simulink model "Task_No6"  (R2023b)
settings: Solver=ode5  StartTime=0.0  StopTime=3600*24*7  FixedStep=1  RelTol=1e-3
InitFcn:
  | PARAMETERS;
StartFcn:
  | PARAMETERS;
values from neighbouring files (symbols this model uses):
  Conv_C_to_K = 273.15    [PARAMETERS.m]
  P_AC_AIR_FLOW = 1    [PARAMETERS.m]
  P_CP_AIR = 1012    [PARAMETERS.m]
  P_DENSITY_AIR = 1.2041    [PARAMETERS.m]
  P_DENSITY_BRICK = 2/(10^-3)    (= 2000)    [PARAMETERS.m]
  P_DENSITY_PUR = 150    [PARAMETERS.m]
  P_EM_GLASS = 0.94    [PARAMETERS.m]
  P_EM_WALL = 0.94    [PARAMETERS.m]
  P_HANDLER_AIR_FLOW = 0.1    [PARAMETERS.m]
  P_HUMAN = 100    [PARAMETERS.m]
  P_INIT_CO2 = 420    [PARAMETERS.m]
  P_M_HUMAN_CO2 = 0.02*P_DENSITY_CO2/3600    (= 1.1e-05)    [PARAMETERS.m]
  P_M_HUMAN_VAPOR = 500*10^-3/(24*3600)    (= 5.78703703704e-06)    [PARAMETERS.m]
  P_M_WINDOW_SPEC = 20    [PARAMETERS.m]
  P_THICK_BRICK = 0.175    [PARAMETERS.m]
  P_THICK_PUR = P_THICK_WALL - P_THICK_BRICK    (= 0.125)    [PARAMETERS.m]
  RH_INIT_BDR = 40    [PARAMETERS.m]
  T_BREATH = 34    [PARAMETERS.m]
  T_COOLER = 12    [PARAMETERS.m]
  T_HEATER = 50    [PARAMETERS.m]
  T_INIT_BDR = 22    [PARAMETERS.m]
  T_INIT_OUT = 2.9    [PARAMETERS.m]
  U_WALL = 0.32    [PARAMETERS.m]
  U_WINDOW = 3.0    (= 3)    [PARAMETERS.m]
undefined symbols (not defined in the file or in its folder): P_AREA_BATH, P_AREA_BDR1, P_AREA_BDR2, P_AREA_EAST_WALL_BATH, P_AREA_EAST_WALL_BDR2, P_AREA_EAST_WALL_KIT, P_AREA_HALL, P_AREA_KIT, P_AREA_LVR, P_AREA_NORTH_WALL_BATH, P_AREA_NORTH_WALL_BDR1, P_AREA_NORTH_WALL_BDR2, P_AREA_OUTER_WALL_BATH, P_AREA_OUTER_WALL_BDR1, P_AREA_OUTER_WALL_BDR2, P_AREA_OUTER_WALL_HALL, P_AREA_OUTER_WALL_KIT, P_AREA_OUTER_WALL_LVR, P_AREA_SOUTH_WALL_KIT, P_AREA_SOUTH_WALL_LVR, P_AREA_WALL_BATH_KIT, P_AREA_WALL_BDR1_BDR2, P_AREA_WALL_BDR1_HALL, P_AREA_WALL_BDR2_BATH, P_AREA_WALL_BDR2_HALL, P_AREA_WALL_HALL_BATH, P_AREA_WALL_HALL_LVR, P_AREA_WALL_LVR_KIT, P_AREA_WIN_BATH, P_AREA_WIN_BDRS, P_AREA_WIN_KIT, P_AREA_WIN_LVR, P_M_AIR_BATH, P_M_AIR_BDR1, P_M_AIR_BDR2, P_M_AIR_HALL, P_M_AIR_KIT, P_M_AIR_LVR, TBL_SOL_EAST_01, TBL_SOL_EAST_02, TBL_SOL_EAST_03, TBL_SOL_EAST_04, TBL_SOL_EAST_05, TBL_SOL_EAST_06, TBL_SOL_EAST_07, TBL_SOL_EAST_08, TBL_SOL_EAST_09, TBL_SOL_EAST_10, TBL_SOL_EAST_11, TBL_SOL_EAST_12, TBL_SOL_NORTH_01, TBL_SOL_NORTH_02, TBL_SOL_NORTH_03, TBL_SOL_NORTH_04, TBL_SOL_NORTH_05, TBL_SOL_NORTH_06, TBL_SOL_NORTH_07, TBL_SOL_NORTH_08, TBL_SOL_NORTH_09, TBL_SOL_NORTH_10 ... (+7)
libraries: fl_lib x166, nesl_utility x88, slpidlib x3
(part 1 of 5)
settings Model: Creator=Selim  LastModifiedBy=Selim

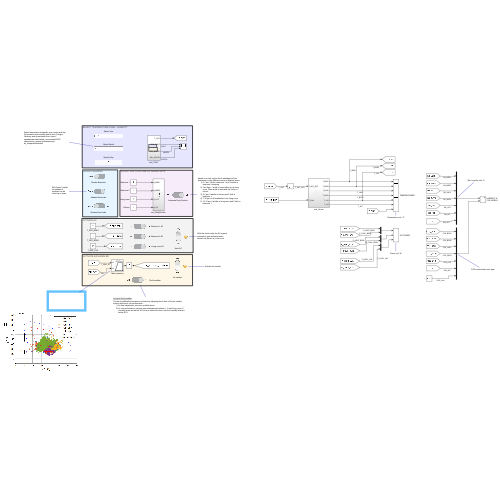
[thumbnail: Simulink's stored preview of the top-level diagram]
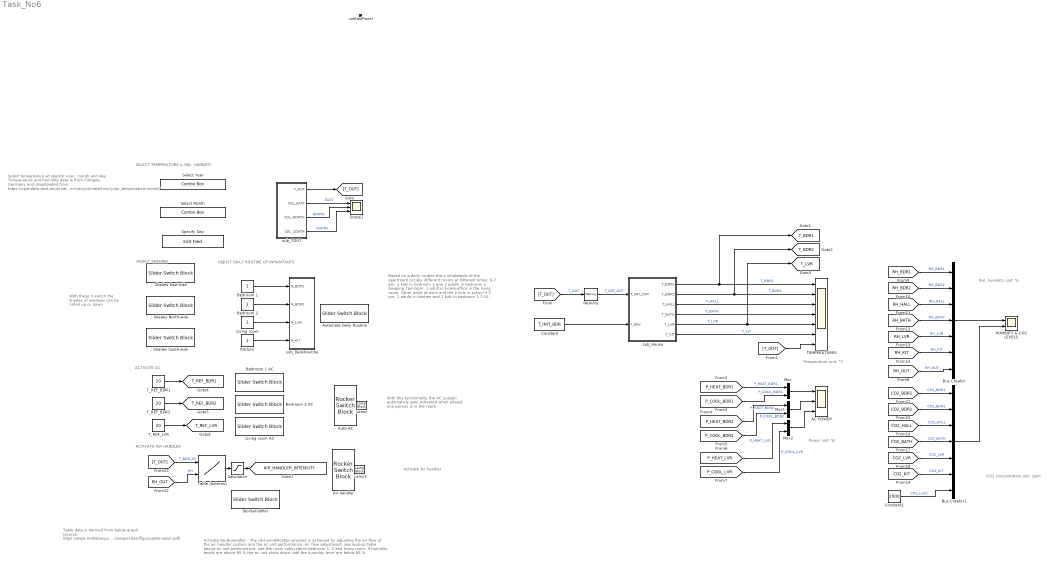
== system Task_No6 ==
  note: Table data is derived from below graph (source: https://www.matlabexpo.com/content/dam/mathworks/mathworks-dot-com/images/events/matlabexpo/de/2017/gebaude-und-anlagensimulation-mit-matlab-und-simulink-am-beispiel-des-ffg-projekts-saluh.pdf)
  note: Activate De-Humidifier :
      | The de-humidification process is achieved by adjusting the air flow of the air handler system and the ac unit performance.
      | Air flow adjustment: see look-up table above
      | Ac unit performance: see the room subsystems bedroom 1, 2 and living room. If humidity levels are above 85 % the ac unit shuts down until the humidity level are below 85 %.
  note: Activate Air handler
  note: Select temperature at specific year, month and day. Temperature and humidity data is from Cologne, Germany and downloaded from: https://opendata.dwd.de/climate_environment/CDC/observations_germany/climate/hourly/air_temperature/recent/
  note: ACTIVATE AIR HANDLER
  note: ACTIVATE AC
  note: ADJUST DAILY ROUTINE OF INHABITANTS
  note: ADJUST SHADING
  note: With these 3 switch the shades of windows can be rolled up or down
  note: CO2 concentration unit: ppm
  note: Rel. humidity unit: %
  note: Temperature unit: °C
  note: With this functionality the AC system automaticly gets activated when atleast one person is in the room
  note: SELECT TEMPERATURE & REL. HUMIDITY
  note: Based on a daily routine the 4 inhabitants of the apartment occupy different rooms at different times:
      | 0-7 am: 2 kids in bedroom 1 and 2 adults in bedroom 2 sleeping
      | 7am-5pm: 1 adult in home-office in the living room. Other adult at work and the 2 kids in school
      | 5-7 pm: 2 adults in kitchen and 2 kids in bedroom 1
      | 7-10 pm: all 4 inhabitants in the living room
      | 10-12 pm: 2 adults in living room and 2 kids in bedroom 1
  note: Power unit: W
  AC POWER : Scope  NumInputPorts=3
  Air handler : RockerSwitchBlock  LabelPosition=Hide
      settings: Values={{'Off', 'On'}, [0 1]}
  Auto-AC : RockerSwitchBlock  LabelPosition=Hide
      settings: Values={{'Off', 'On'}, [0 1]}
  Automate Daily Routine : SliderSwitchBlock  LabelPosition=Hide
      settings: Values={{'OFF', 'ON'}, [0 1]}
  Bedroom 1 : Constant
  Bedroom 1 AC : SliderSwitchBlock  LabelPosition=Hide
      settings: Values={{'OFF', 'ON'}, [0 1]}
  Bedroom 2 : Constant
  Bedroom 2 AC : SliderSwitchBlock  LabelPosition=Hide
      settings: Values={{'OFF', 'ON'}, [0 1]}
  Bus Creator : BusCreator  Inputs=7
  Bus Creator1 : BusCreator  Inputs=7
  Constant : Constant  Value=T_INIT_BDR
  Constant1 : Constant  Value=2000
  De-Humidifier : SliderSwitchBlock  LabelPosition=Hide
      settings: Values={{'OFF', 'ON'}, [0 1]}
  HUMIDITY & CO2 LEVELS : Scope  NumInputPorts=2
  Kitchen : Constant
  Lamp : LampBlock  LabelPosition=Hide
  Lamp1 : LampBlock  LabelPosition=Hide
  Living room : Constant
  Living room AC : SliderSwitchBlock  LabelPosition=Hide
      settings: Values={{'OFF', 'ON'}, [0 1]}
  Memory : Memory  InitialCondition=T_INIT_OUT
  Mux : Mux  Inputs=2
  Mux1 : Mux  Inputs=2
  Mux2 : Mux  Inputs=2
  Saturation : Saturate  UpperLimit=inf  LowerLimit=0
  Scope1 : Scope  NumInputPorts=3
  Select Month : ComboBox  LabelPosition=Hide  SelectedLabel=July
      settings: Values={{'January', 'February', 'March', 'April', 'May', 'June', 'July', 'August', 'September', 'Oktober', 'November', 'December'}, [1 2 3 4 5 6 7 8 9 10 11 12]}
  Select Year : ComboBox  LabelPosition=Hide  SelectedLabel=2023
      settings: Values={{'2022', '2023'}, [2022 2023]}
  Shades East-side : SliderSwitchBlock  LabelPosition=Hide
      settings: Values={{'Down', 'Up'}, [0 1]}
  Shades North-side : SliderSwitchBlock  LabelPosition=Hide
      settings: Values={{'Down', 'Up'}, [0 1]}
  Shades South-side : SliderSwitchBlock  LabelPosition=Hide
      settings: Values={{'Down', 'Up'}, [0 1]}
  Specify Day : EditField  LabelPosition=Hide  ShowInitialText=on  Alignment=Center
  TEMPERATURES : Scope  NumInputPorts=7
  T_REF_BDR1 : Constant  Value=20
  T_REF_BDR2 : Constant  Value=20
  T_REF_LVR : Constant  Value=20
  Table (exterior) : Lookup_n-D  BreakpointsForDimension1=[16;19;24;24.5]  BreakpointsForDimension2=[20;25;58;82]  Table=[0.5 0.5 0.5 0.5;0.5 1 1 0.5;0.5 1 1 0.5;0.5 0.5 0.5 0.5]  ExtrapMethod=Clip  InternalRulePriority=Speed  RndMeth=Simplest
      settings: InputPortMap=u0,u1
  sub_DailyRoutine : Subsystem
  sub_House : Subsystem
  sub_TOUT : Subsystem
  untitledPanel : Subsystem  Tag=HiddenForWebPanel  IsWebBlockPanel=on
  tag scope: AIR_HANDLER_INTENSITY=global, T_BDR1=global, T_BDR2=global, T_LVR=global, T_REF_BDR1=global, T_REF_BDR2=global, T_REF_LVR=global
  wires:
  Memory/1 -> sub_House/1(T_INIT_OUT)  "T_INIT_OUT"
  sub_House/1(T_BDR1) -> [T_BDR1], TEMPERATURES/1  "T_BDR1"
  [T_OUT] -> Memory/1  "T_OUT"
  [T_OUT] -> TEMPERATURES/7
  Constant/1 -> sub_House/2(T_ENV)
  sub_TOUT/1(T_OUT) -> [T_OUT]
  sub_House/2(T_BDR2) -> [T_BDR2], TEMPERATURES/2  "T_BDR2"
  sub_House/3(T_HALL) -> TEMPERATURES/3  "T_HALL"
  sub_House/4(T_BATH) -> TEMPERATURES/4  "T_BATH"
  sub_House/5(T_LVR) -> [T_LVR], TEMPERATURES/5  "T_LVR"
  sub_House/6(T_KIT) -> TEMPERATURES/6  "T_KIT"
  sub_TOUT/2(SOL_EAST) -> Scope1/1  "EAST"
  sub_TOUT/3(SOL_NORTH) -> Scope1/2  "NORTH"
  sub_TOUT/4(SOL_SOUTH) -> Scope1/3  "SOUTH"
  Bedroom 1/1 -> sub_DailyRoutine/1(N_BDR1)
  Bedroom 2/1 -> sub_DailyRoutine/2(N_BDR2)
  Living room/1 -> sub_DailyRoutine/3(N_LVR)
  Kitchen/1 -> sub_DailyRoutine/4(N_KIT)
  T_REF_BDR1/1 -> [T_REF_BDR1]
  T_REF_BDR2/1 -> [T_REF_BDR2]
  T_REF_LVR/1 -> [T_REF_LVR]
  Mux/1 -> AC POWER/1
  Mux1/1 -> AC POWER/2
  Mux2/1 -> AC POWER/3
  [P_HEAT_BDR1] -> Mux/1  "P_HEAT_BDR1"
  [P_COOL_BDR1] -> Mux/2  "P_COOL_BDR1"
  [P_HEAT_BDR2] -> Mux1/1  "P_HEAT_BDR2"
  [P_COOL_BDR2] -> Mux1/2  "P_COOL_BDR2"
  [P_HEAT_LVR] -> Mux2/1  "P_HEAT_LVR"
  [P_COOL_LVR] -> Mux2/2  "P_COOL_LVR"
  [RH_BDR1] -> Bus Creator/1  "RH_BDR1"
  [RH_BDR2] -> Bus Creator/2  "RH_BDR2"
  [RH_HALL] -> Bus Creator/3  "RH_HALL"
  [RH_BATH] -> Bus Creator/4  "RH_BATH"
  [RH_LVR] -> Bus Creator/5  "RH_LVR"
  [RH_KIT] -> Bus Creator/6  "RH_KIT"
  [RH_OUT] -> Bus Creator/7  "RH_OUT"
  [CO2_BDR1] -> Bus Creator1/1  "CO2_BDR1"
  [CO2_BDR2] -> Bus Creator1/2  "CO2_BDR2"
  [CO2_HALL] -> Bus Creator1/3  "CO2_HALL"
  [CO2_BATH] -> Bus Creator1/4  "CO2_BATH"
  [CO2_LVR] -> Bus Creator1/5  "CO2_LVR"
  [CO2_KIT] -> Bus Creator1/6  "CO2_KIT"
  Bus Creator/1 -> HUMIDITY & CO2 LEVELS/1
  Bus Creator1/1 -> HUMIDITY & CO2 LEVELS/2
  Constant1/1 -> Bus Creator1/7  "CO2_Limit"
  Table (exterior)/1 -> Saturation/1
  [T_OUT] -> Table (exterior)/1  "T_BDR_SC"
  [RH_OUT] -> Table (exterior)/2  "RH"
  Saturation/1 -> [AIR_HANDLER_INTENSITY]

== system Task_No6/sub_DailyRoutine ==
  N_BDR1 : Inport
  N_BDR2 : Inport  Port=2
  N_LVR : Inport  Port=3
  N_KIT : Inport  Port=4
  DAILY_ROUTINE_ON : Constant
  Memory1 : Memory
  Switch{,1..3} (4 alike) : Switch  Criteria=u2 > Threshold  SaturateOnIntegerOverflow=off  InputSameDT=off
  Time of day : MATLAB Function  TreatAsAtomicUnit=on
  tag scope: N_BDR1=global, N_BDR2=global, N_KIT=global, N_LVR=global
  wires:
  Switch1/1 -> [N_BDR2]
  Switch2/1 -> [N_LVR]
  Time of day/1(h) -> Memory1/1
  Memory1/1 -> Time of day/1("h ")
  Switch/1 -> [N_BDR1]
  Switch3/1 -> [N_KIT]
  Time of day/2(n_bdr1) -> Switch/1
  Time of day/3(n_bdr2) -> Switch1/1
  Time of day/4(n_lvr) -> Switch2/1
  Time of day/5(n_kit) -> Switch3/1
  DAILY_ROUTINE_ON/1 -> Switch3/2, Switch2/2, Switch1/2, Switch/2
  N_BDR1/1 -> Switch/3
  N_BDR2/1 -> Switch1/3
  N_LVR/1 -> Switch2/3
  N_KIT/1 -> Switch3/3

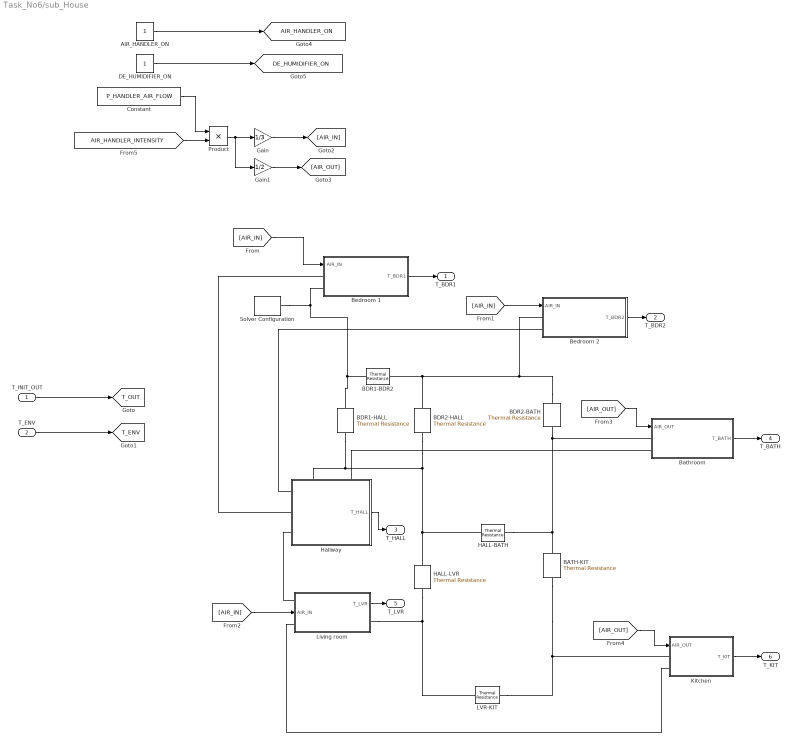
== system Task_No6/sub_House ==
  T_INIT_OUT : Inport
  T_ENV : Inport  Port=2
  AIR_HANDLER_ON : Constant
  BATH-KIT : fl_lib/Thermal/Thermal Elements/Thermal Resistance  resistance=1/(U_INNER_WALL_PC*P_AREA_WALL_BATH_KIT) K/W  T_specify=off  T_priority=None  T=0 K  T_nominal_specify=off  T_nominal_unit=K  T_nominal_value=1  Q_specify=off  Q_priority=None  Q=0 W  Q_nominal_specify=off  Q_nominal_unit=W  Q_nominal_value=1
  BDR1-BDR2 : fl_lib/Thermal/Thermal Elements/Thermal Resistance  resistance=1/(U_INNER_WALL_BR*P_AREA_WALL_BDR1_BDR2) K/W  T_specify=off  T_priority=None  T=0 K  T_nominal_specify=off  T_nominal_unit=K  T_nominal_value=1  Q_specify=off  Q_priority=None  Q=0 W  Q_nominal_specify=off  Q_nominal_unit=W  Q_nominal_value=1
  BDR1-HALL : fl_lib/Thermal/Thermal Elements/Thermal Resistance  resistance=1/(U_INNER_WALL_PC*P_AREA_WALL_BDR1_HALL) K/W  T_specify=off  T_priority=None  T=0 K  T_nominal_specify=off  T_nominal_unit=K  T_nominal_value=1  Q_specify=off  Q_priority=None  Q=0 W  Q_nominal_specify=off  Q_nominal_unit=W  Q_nominal_value=1
  BDR2-BATH : fl_lib/Thermal/Thermal Elements/Thermal Resistance  resistance=1/(U_INNER_WALL_PC*P_AREA_WALL_BDR2_BATH) K/W  T_specify=off  T_priority=None  T=0 K  T_nominal_specify=off  T_nominal_unit=K  T_nominal_value=1  Q_specify=off  Q_priority=None  Q=0 W  Q_nominal_specify=off  Q_nominal_unit=W  Q_nominal_value=1
  BDR2-HALL : fl_lib/Thermal/Thermal Elements/Thermal Resistance  resistance=1/(U_INNER_WALL_PC*P_AREA_WALL_BDR2_HALL) K/W  T_specify=off  T_priority=None  T=0 K  T_nominal_specify=off  T_nominal_unit=K  T_nominal_value=1  Q_specify=off  Q_priority=None  Q=0 W  Q_nominal_specify=off  Q_nominal_unit=W  Q_nominal_value=1
  Bathroom : Subsystem
  Bedroom 1 : Subsystem
  Bedroom 2 : Subsystem
  Constant : Constant  Value=P_HANDLER_AIR_FLOW
  DE_HUMIDIFIER_ON : Constant
  Gain : Gain  Gain=1/3
  Gain1 : Gain  Gain=1/2
  HALL-BATH : fl_lib/Thermal/Thermal Elements/Thermal Resistance  resistance=1/(U_INNER_WALL_BR*P_AREA_WALL_HALL_BATH) K/W  T_specify=off  T_priority=None  T=0 K  T_nominal_specify=off  T_nominal_unit=K  T_nominal_value=1  Q_specify=off  Q_priority=None  Q=0 W  Q_nominal_specify=off  Q_nominal_unit=W  Q_nominal_value=1
  HALL-LVR : fl_lib/Thermal/Thermal Elements/Thermal Resistance  resistance=1/(U_INNER_WALL_PC*P_AREA_WALL_HALL_LVR) K/W  T_specify=off  T_priority=None  T=0 K  T_nominal_specify=off  T_nominal_unit=K  T_nominal_value=1  Q_specify=off  Q_priority=None  Q=0 W  Q_nominal_specify=off  Q_nominal_unit=W  Q_nominal_value=1
  Hallway : Subsystem
      settings: PortSchema="{\"entries\":[{\"content\":{\"sides\":[{\"content\":{\"connectorIds\":[\"LConn1\",\"LConn2\",\"LConn3\"]},\"type\":\"ConnectorPlacement.EquallySpacedRectSide\",\"uuid\":\"489b9df6-19cb-4475-a274-302d4b8f34a0\"},{\"content\":{\"connectorIds\":[\"Out1\"],\"side\":\"RIGHT\"},\"type\":\"ConnectorPlacement.EquallySpacedRectSide\",\"uuid\":\"503e44aa-58ca-4784-9bf5-a317de849747\"},{\"content\":{\"connectorIds\":[\"LConn4\",\"LConn5\"],\"side\":\"TOP\"},\"type\":\"ConnectorPlacement.EquallySpacedRectSide\",\"uuid\":\"5734f698-8762-4391-9ecf-ea0e4ab42052\"}]},\"type\":\"ConnectorPlacement.EquallySpacedConnector\",\"uuid\":\"2aa354c6-d8ba-4f9b-b434-ff0d4333e4a9\"}],\"packageUris\":[\"http://schema.mathworks.com/mf0/Connector/R2020b\"],\"version\":\"1.0\"}"
  Kitchen : Subsystem
  LVR-KIT : fl_lib/Thermal/Thermal Elements/Thermal Resistance  resistance=1/(U_INNER_WALL_BR*P_AREA_WALL_LVR_KIT) K/W  T_specify=off  T_priority=None  T=0 K  T_nominal_specify=off  T_nominal_unit=K  T_nominal_value=1  Q_specify=off  Q_priority=None  Q=0 W  Q_nominal_specify=off  Q_nominal_unit=W  Q_nominal_value=1
  Living room : Subsystem
      settings: PortSchema="{\"entries\":[{\"content\":{\"sides\":[{\"content\":{\"connectorIds\":[\"LConn1\",\"In1\",\"LConn2\"]},\"type\":\"ConnectorPlacement.EquallySpacedRectSide\",\"uuid\":\"f71185e0-26fc-428d-a49e-eba48eb4716b\"},{\"content\":{\"connectorIds\":[\"Out1\",\"RConn1\"],\"side\":\"RIGHT\"},\"type\":\"ConnectorPlacement.EquallySpacedRectSide\",\"uuid\":\"b5ccd292-c29d-4ca4-a01f-fb6127cce0f9\"},{\"content\":{\"side\":\"TOP\"},\"type\":\"ConnectorPlacement.EquallySpacedRectSide\",\"uuid\":\"45f0e2e7-39cb-4c88-b766-6fb6aae0cec8\"}]},\"type\":\"ConnectorPlacement.EquallySpacedConnector\",\"uuid\":\"6a8451ab-eb03-49e5-afa1-3415116fa991\"}],\"packageUris\":[\"http://schema.mathworks.com/mf0/Connector/R2020b\"],\"version\":\"1.0\"}"
  Product : Product
  Solver Configuration : nesl_utility/Solver Configuration  PhysicalDomain=network_engine_domain  SubClassName=solver  LeftPortType=input  RightPortType=generic  Tones=[]  Harmonics=[]  SimulateNoise=off  Profile=off  UseLocalSampling=off  EnableSwitchedLinearOptims=on  FrequencyDomain=off  UseCCode=off  RelTol=0.001  AbsTol=0.001  MinStep=1e-09  ToWorkspace=off  RevertToSquareIcSolve=off  NumHomotopyIterations=100  PhasorMode=off  PhasorModeNumHarmonics=1  ConsistencySolver=NEWTON_XTOL_AFTER_FTOL  IndexReductionMethod=DerivativeReplacement  DoDC=off  ResidualTolerance=1e-09  ConsistencyTolSource=GLOBAL  ConsistencyAbsTol=0.001  ConsistencyRelTol=0.001  ConsistencyTolFactor=0.001  UseLocalSolver=on  LocalSolverChoice=NE_BACKWARD_EULER_ADVANCER  ResolveIndetEquations=on  FunctionEvalNumThread=1  LocalSolverSampleTime=1  DoFixedCost=on  MaxNonlinIter=3  MaxModeIter=2  ComputeImpulses=off  ImpulseIterations=2  LinearAlgebra=auto  LinearAlgebraNumThread=0  EquationFormulation=NE_TIME_EF  DelaysMemoryBudget=1024  AutomaticFiltering=on  FilteringTimeConstant=0.001  PartitionStorageMethod=AS_NEEDED  PartitionMemoryBudget=1024  PartitionMethod=ROBUST  MultibodyUseLocalSolver=off  MultibodyLocalSolverChoice=ODE1  MultibodyLocalSolverSampleTime=0.001
  T_BDR1 : Outport
  T_BDR2 : Outport  Port=2
  T_HALL : Outport  Port=3
  T_BATH : Outport  Port=4
  T_LVR : Outport  Port=5
  T_KIT : Outport  Port=6
  tag scope: AIR_HANDLER_ON=global, DE_HUMIDIFIER_ON=global, T_ENV=global, T_OUT=global
  wires:
  T_INIT_OUT/1 -> [T_OUT]
  T_ENV/1 -> [T_ENV]
  Bedroom 1/1(T_BDR1) -> T_BDR1/1
  Bedroom 2/1(T_BDR2) -> T_BDR2/1
  Hallway/1(T_HALL) -> T_HALL/1
  Living room/1(T_LVR) -> T_LVR/1
  Bathroom/1(T_BATH) -> T_BATH/1
  Kitchen/1(T_KIT) -> T_KIT/1
  Constant/1 -> Product/1
  Gain/1 -> [AIR_IN]
  [AIR_IN] -> Bedroom 1/1(AIR_IN)
  [AIR_IN] -> Bedroom 2/1(AIR_IN)
  [AIR_IN] -> Living room/1(AIR_IN)
  Gain1/1 -> [AIR_OUT]
  [AIR_OUT] -> Bathroom/1(AIR_OUT)
  [AIR_OUT] -> Kitchen/1(AIR_OUT)
  AIR_HANDLER_ON/1 -> [AIR_HANDLER_ON]
  [AIR_HANDLER_INTENSITY] -> Product/2
  Product/1 -> Gain/1, Gain1/1
  DE_HUMIDIFIER_ON/1 -> [DE_HUMIDIFIER_ON]
  connections:
  Solver Configuration/RConn1 -- BDR1-HALL/LConn1 -- BDR1-BDR2/RConn1 -- Bedroom 1/LConn2
  BDR2-BATH/LConn1 -- Bedroom 2/LConn1 -- BDR2-HALL/LConn1 -- BDR1-BDR2/LConn1
  BDR2-BATH/RConn1 -- HALL-BATH/LConn1 -- BATH-KIT/LConn1 -- Bathroom/LConn1
  HALL-LVR/RConn1 -- LVR-KIT/RConn1 -- Living room/RConn1
  BDR1-HALL/RConn1 -- HALL-LVR/LConn1 -- HALL-BATH/RConn1 -- BDR2-HALL/RConn1 -- Hallway/LConn4
  Hallway/LConn2 -- Bedroom 1/LConn1
  Hallway/LConn1 -- Bedroom 2/LConn2
  Living room/LConn1 -- Hallway/LConn3
  Hallway/LConn5 -- Bathroom/LConn2
  BATH-KIT/RConn1 -- LVR-KIT/LConn1 -- Kitchen/LConn1
  Kitchen/LConn2 -- Living room/LConn2

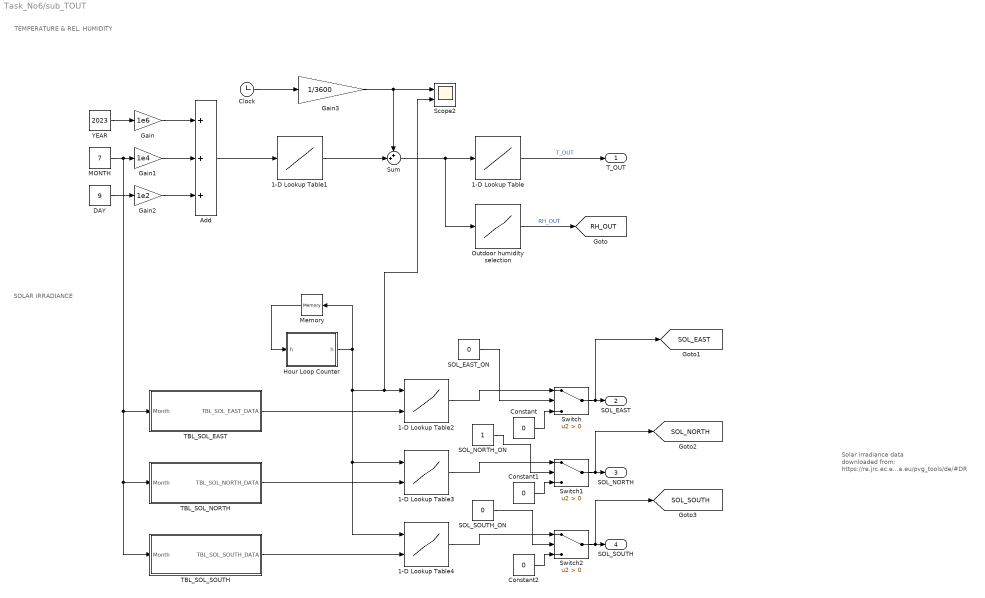
== system Task_No6/sub_TOUT ==
  note: Solar irradiance data downloaded from: https://re.jrc.ec.europa.eu/pvg_tools/de/#DR
  note: SOLAR IRRADIANCE
  note: TEMPERATURE & REL. HUMIDITY
  1-D Lookup Table : Lookup_n-D  NumberOfTableDimensions=1  BreakpointsForDimension1=TBL_TEMP.DATE_sec  Table=TBL_TEMP.T_C  InternalRulePriority=Speed  RndMeth=Simplest
  1-D Lookup Table1 : Lookup_n-D  NumberOfTableDimensions=1  BreakpointsForDimension1=TBL_TEMP.DATE_yyyymmddhh  Table=TBL_TEMP.DATE_sec  InternalRulePriority=Speed  RndMeth=Simplest
  1-D Lookup Table2 : Lookup_n-D  NumberOfTableDimensions=1  BreakpointsForDimension1=0:1:23  TableSource=Input port  Table=tanh([-5:5])  InternalRulePriority=Speed  RndMeth=Simplest
      settings: InputPortMap=u0,p221
  1-D Lookup Table3 : Lookup_n-D  NumberOfTableDimensions=1  BreakpointsForDimension1=0:1:23  TableSource=Input port  Table=tanh([-5:5])  InternalRulePriority=Speed  RndMeth=Simplest
      settings: InputPortMap=u0,p221
  1-D Lookup Table4 : Lookup_n-D  NumberOfTableDimensions=1  BreakpointsForDimension1=0:1:23  TableSource=Input port  Table=tanh([-5:5])  InternalRulePriority=Speed  RndMeth=Simplest
      settings: InputPortMap=u0,p221
  Add : Sum  Inputs=+++
  Clock : Clock
  Constant : Constant  Value=0
  Constant1 : Constant  Value=0
  Constant2 : Constant  Value=0
  DAY : Constant  Value=9
  Gain : Gain  Gain=1e6
  Gain1 : Gain  Gain=1e4
  Gain2 : Gain  Gain=1e2
  Gain3 : Gain  Gain=1/3600
  Hour Loop Counter : MATLAB Function  TreatAsAtomicUnit=on
  MONTH : Constant  Value=7
  Memory : Memory
  Outdoor humidity selection : Lookup_n-D  NumberOfTableDimensions=1  BreakpointsForDimension1=TBL_TEMP.DATE_sec  Table=TBL_TEMP.RM_p100  InternalRulePriority=Speed  RndMeth=Simplest
  SOL_EAST_ON : Constant  Value=0
  SOL_NORTH_ON : Constant
  SOL_SOUTH_ON : Constant  Value=0
  Scope2 : Scope  NumInputPorts=2
  Sum : Sum  Inputs=++|
  Switch : Switch  Criteria=u2 > Threshold  SaturateOnIntegerOverflow=off  InputSameDT=off
  Switch1 : Switch  Criteria=u2 > Threshold  SaturateOnIntegerOverflow=off  InputSameDT=off
  Switch2 : Switch  Criteria=u2 > Threshold  SaturateOnIntegerOverflow=off  InputSameDT=off
  TBL_SOL_EAST : Subsystem
  TBL_SOL_NORTH : Subsystem
  TBL_SOL_SOUTH : Subsystem
  YEAR : Constant  Value=2023
  T_OUT : Outport
  SOL_EAST : Outport  Port=2
  SOL_NORTH : Outport  Port=3
  SOL_SOUTH : Outport  Port=4
  tag scope: RH_OUT=global, SOL_EAST=global, SOL_NORTH=global, SOL_SOUTH=global
  wires:
  Gain1/1 -> Add/2
  MONTH/1 -> TBL_SOL_SOUTH/1(Month), TBL_SOL_NORTH/1(Month), TBL_SOL_EAST/1(Month), Gain1/1
  Clock/1 -> Gain3/1
  1-D Lookup Table1/1 -> Sum/2
  Add/1 -> 1-D Lookup Table1/1
  YEAR/1 -> Gain/1
  Gain/1 -> Add/1
  Gain3/1 -> Scope2/1, Sum/1
  Sum/1 -> Outdoor humidity selection/1, 1-D Lookup Table/1
  Gain2/1 -> Add/3
  DAY/1 -> Gain2/1
  1-D Lookup Table/1 -> T_OUT/1  "T_OUT"
  Hour Loop Counter/1(h) -> 1-D Lookup Table4/1, 1-D Lookup Table3/1, Scope2/2, 1-D Lookup Table2/1, Memory/1
  Memory/1 -> Hour Loop Counter/1("h ")
  Switch/1 -> [SOL_EAST], SOL_EAST/1
  TBL_SOL_EAST/1(TBL_SOL_EAST_DATA) -> 1-D Lookup Table2/2
  TBL_SOL_NORTH/1(TBL_SOL_NORTH_DATA) -> 1-D Lookup Table3/2
  TBL_SOL_SOUTH/1(TBL_SOL_SOUTH_DATA) -> 1-D Lookup Table4/2
  Switch1/1 -> [SOL_NORTH], SOL_NORTH/1
  Switch2/1 -> [SOL_SOUTH], SOL_SOUTH/1
  1-D Lookup Table2/1 -> Switch/1
  1-D Lookup Table3/1 -> Switch1/1
  1-D Lookup Table4/1 -> Switch2/1
  SOL_EAST_ON/1 -> Switch/2
  Constant/1 -> Switch/3
  Constant1/1 -> Switch1/3
  Constant2/1 -> Switch2/3
  SOL_NORTH_ON/1 -> Switch1/2
  SOL_SOUTH_ON/1 -> Switch2/2
  Outdoor humidity selection/1 -> [RH_OUT]  "RH_OUT"

== system Task_No6/untitledPanel ==
  Radio Button : RadioButtonGroup  Tag=HiddenForWebPanel  PanelInfo="{\"addnFilesFolder\":\"\",\"height\":230,\"includeDebugPackages\":false,\"left\":18,\"outputFolder\":\"\",\"panelId\":\"panelId-a10107d6-1e7d-451d-956e-0df6eada92c1\",\"popoutMode\":\"\",\"standaloneTitle\":\"\",\"top\":18,\"type\":\"panelChild\",\"version\":\"2019b\",\"width\":270,\"zIndex\":1500002}"  SelectedLabel=Label3  ButtonGroupName=Group
      settings: Values={{'Label1', 'Label2', 'Label3'}, [0 1 2]}
  panelInfo : PanelWebBlock  Tag=HiddenForWebPanel  PanelInfo="{\"addnFilesFolder\":\"\",\"compacted\":false,\"height\":270,\"includeDebugPackages\":false,\"isActiveTab\":true,\"left\":296,\"name\":\"Panel\",\"outputFolder\":\"\",\"panelId\":\"panelId-a10107d6-1e7d-451d-956e-0df6eada92c1\",\"popoutData\":{\"height\":334,\"left\":361,\"maximized\":false,\"top\":306,\"width\":324},\"popoutMode\":\"windowHidden\",\"standaloneTitle\":\"\",\"tabIndex\":0,\"tabbedSetId\":\"tabbedSet8433950298\",\"top\":135,\"type\":\"panel\",\"version\":\"2019b\",\"visible\":true,\"width\":310,\"zIndex\":1500002}"

== system Task_No6/sub_House/Bathroom ==
  AIR_OUT : Inport
  Bathroom : Subsystem
  MA Bathroom : Subsystem
  Product : Product
  Conn1 : PMIOPort  Side=Left
  HALL-BATH : PMIOPort  Port=2  Side=Left
  T_BATH : Outport
  wires:
  AIR_OUT/1 -> Product/1
  Bathroom/1(T_BATH) -> T_BATH/1
  [AIR_HANDLER_ON] -> Product/2
  Product/1 -> MA Bathroom/1(In1)
  connections:
  MA Bathroom/RConn1 -- Conn1/RConn1 -- Bathroom/LConn1
  HALL-BATH/RConn1 -- MA Bathroom/LConn1

== system Task_No6/sub_House/Bedroom 1 ==
  AIR_IN : Inport
  Bedroom 1 : Subsystem
  MA Bedroom 1 : Subsystem
  Product : Product
  BDR1-HALL : PMIOPort  Side=Left
  Conn1 : PMIOPort  Port=2  Side=Left
  T_BDR1 : Outport
  wires:
  AIR_IN/1 -> Product/1
  Bedroom 1/1(T_BDR1) -> T_BDR1/1
  Product/1 -> MA Bedroom 1/1(In1)
  [AIR_HANDLER_ON] -> Product/2
  connections:
  MA Bedroom 1/RConn1 -- Conn1/RConn1 -- Bedroom 1/LConn1
  BDR1-HALL/RConn1 -- MA Bedroom 1/LConn1

== system Task_No6/sub_House/Bedroom 2 ==
  AIR_IN : Inport
  Bedroom 2 : Subsystem
  MA Bedroom 2 : Subsystem
  Product : Product
  Conn1 : PMIOPort  Side=Left
  BDR2-HALL : PMIOPort  Port=2  Side=Left
  T_BDR2 : Outport
  wires:
  Bedroom 2/1(T_BDR2) -> T_BDR2/1
  AIR_IN/1 -> Product/1
  [AIR_HANDLER_ON] -> Product/2
  Product/1 -> MA Bedroom 2/1(In1)
  connections:
  BDR2-HALL/RConn1 -- MA Bedroom 2/LConn1
  MA Bedroom 2/RConn1 -- Conn1/RConn1 -- Bedroom 2/LConn1

== system Task_No6/sub_House/Hallway ==
  Hallway : Subsystem
  MA Hallway : Subsystem
  BDR2-HALL : PMIOPort  Side=Left
  BDR1-HALL : PMIOPort  Port=2  Side=Left
  LVR-HALL : PMIOPort  Port=3  Side=Left
  Conn4 : PMIOPort  Port=4  Side=Left
  HALL-BATH : PMIOPort  Port=5  Side=Left
  T_HALL : Outport
  wires:
  Hallway/1(T_HALL) -> T_HALL/1
  connections:
  MA Hallway/LConn4 -- HALL-BATH/RConn1
  Conn4/RConn1 -- MA Hallway/RConn1 -- Hallway/LConn1
  MA Hallway/LConn2 -- BDR1-HALL/RConn1
  MA Hallway/LConn1 -- BDR2-HALL/RConn1
  LVR-HALL/RConn1 -- MA Hallway/LConn3

== system Task_No6/sub_House/Kitchen ==
  AIR_OUT : Inport
  Kitchen : Subsystem
  MA Kitchen : Subsystem
  Product : Product
  Conn1 : PMIOPort  Side=Left
  LVR-KIT : PMIOPort  Port=2  Side=Left
  T_KIT : Outport
  wires:
  AIR_OUT/1 -> Product/1
  Kitchen/1(T_KIT) -> T_KIT/1
  Product/1 -> MA Kitchen/1(In1)
  [AIR_HANDLER_ON] -> Product/2
  connections:
  MA Kitchen/LConn1 -- LVR-KIT/RConn1
  Conn1/RConn1 -- MA Kitchen/RConn1 -- Kitchen/LConn1

== system Task_No6/sub_House/Living room ==
  AIR_IN : Inport
  Living Room : Subsystem
  MA Living Room : Subsystem
  Product : Product
  LVR-HALL : PMIOPort  Side=Left
  LVR-KIT : PMIOPort  Port=2  Side=Left
  Conn2 : PMIOPort  Port=3  Side=Right
  T_LVR : Outport
  wires:
  AIR_IN/1 -> Product/1
  Living Room/1(T_LVR) -> T_LVR/1
  [AIR_HANDLER_ON] -> Product/2
  Product/1 -> MA Living Room/1(In1)
  connections:
  LVR-KIT/RConn1 -- MA Living Room/LConn2
  Conn2/RConn1 -- Living Room/LConn1 -- MA Living Room/RConn1
  MA Living Room/LConn1 -- LVR-HALL/RConn1

== system Task_No6/sub_TOUT/TBL_SOL_EAST ==
  Month : Inport
  Constant : Constant  Value=TBL_SOL_EAST_01.G
  Constant1 : Constant  Value=TBL_SOL_EAST_02.G
  Constant10 : Constant  Value=TBL_SOL_EAST_11.G
  Constant11 : Constant  Value=TBL_SOL_EAST_12.G
  Constant2 : Constant  Value=TBL_SOL_EAST_03.G
  Constant3 : Constant  Value=TBL_SOL_EAST_04.G
  Constant4 : Constant  Value=TBL_SOL_EAST_05.G
  Constant5 : Constant  Value=TBL_SOL_EAST_06.G
  Constant6 : Constant  Value=TBL_SOL_EAST_07.G
  Constant7 : Constant  Value=TBL_SOL_EAST_08.G
  Constant8 : Constant  Value=TBL_SOL_EAST_09.G
  Constant9 : Constant  Value=TBL_SOL_EAST_10.G
  Multiport Switch : MultiPortSwitch  Inputs=12  SaturateOnIntegerOverflow=off  InputSameDT=off
  TBL_SOL_EAST_DATA : Outport
  wires:
  Constant1/1 -> Multiport Switch/3
  Constant5/1 -> Multiport Switch/7
  Constant6/1 -> Multiport Switch/8
  Constant3/1 -> Multiport Switch/5
  Multiport Switch/1 -> TBL_SOL_EAST_DATA/1
  Constant11/1 -> Multiport Switch/13
  Constant/1 -> Multiport Switch/2
  Constant2/1 -> Multiport Switch/4
  Constant7/1 -> Multiport Switch/9
  Constant4/1 -> Multiport Switch/6
  Constant10/1 -> Multiport Switch/12
  Constant9/1 -> Multiport Switch/11
  Constant8/1 -> Multiport Switch/10
  Month/1 -> Multiport Switch/1

== system Task_No6/sub_TOUT/TBL_SOL_NORTH ==
  Month : Inport
  Constant : Constant  Value=TBL_SOL_NORTH_01.G
  Constant1 : Constant  Value=TBL_SOL_NORTH_02.G
  Constant10 : Constant  Value=TBL_SOL_NORTH_11.G
  Constant11 : Constant  Value=TBL_SOL_NORTH_12.G
  Constant2 : Constant  Value=TBL_SOL_NORTH_03.G
  Constant3 : Constant  Value=TBL_SOL_NORTH_04.G
  Constant4 : Constant  Value=TBL_SOL_NORTH_05.G
  Constant5 : Constant  Value=TBL_SOL_NORTH_06.G
  Constant6 : Constant  Value=TBL_SOL_NORTH_07.G
  Constant7 : Constant  Value=TBL_SOL_NORTH_08.G
  Constant8 : Constant  Value=TBL_SOL_NORTH_09.G
  Constant9 : Constant  Value=TBL_SOL_NORTH_10.G
  Multiport Switch : MultiPortSwitch  Inputs=12  SaturateOnIntegerOverflow=off  InputSameDT=off
  TBL_SOL_NORTH_DATA : Outport
  wires:
  Month/1 -> Multiport Switch/1
  Constant8/1 -> Multiport Switch/10
  Constant9/1 -> Multiport Switch/11
  Constant10/1 -> Multiport Switch/12
  Constant4/1 -> Multiport Switch/6
  Constant7/1 -> Multiport Switch/9
  Constant2/1 -> Multiport Switch/4
  Constant/1 -> Multiport Switch/2
  Constant11/1 -> Multiport Switch/13
  Multiport Switch/1 -> TBL_SOL_NORTH_DATA/1
  Constant3/1 -> Multiport Switch/5
  Constant6/1 -> Multiport Switch/8
  Constant5/1 -> Multiport Switch/7
  Constant1/1 -> Multiport Switch/3

== system Task_No6/sub_TOUT/TBL_SOL_SOUTH ==
  Month : Inport
  Constant{,1..11} (12 alike) : Constant  Value=TBL_SOL_SOUTH_01.G
  Multiport Switch : MultiPortSwitch  Inputs=12  SaturateOnIntegerOverflow=off  InputSameDT=off
  TBL_SOL_SOUTH_DATA : Outport
  wires:
  Constant1/1 -> Multiport Switch/3
  Constant5/1 -> Multiport Switch/7
  Constant6/1 -> Multiport Switch/8
  Constant3/1 -> Multiport Switch/5
  Multiport Switch/1 -> TBL_SOL_SOUTH_DATA/1
  Constant11/1 -> Multiport Switch/13
  Constant/1 -> Multiport Switch/2
  Constant2/1 -> Multiport Switch/4
  Constant7/1 -> Multiport Switch/9
  Constant4/1 -> Multiport Switch/6
  Constant10/1 -> Multiport Switch/12
  Constant9/1 -> Multiport Switch/11
  Constant8/1 -> Multiport Switch/10
  Month/1 -> Multiport Switch/1

== system Task_No6/sub_House/Bathroom/Bathroom ==
  Ceiling & Floor (Bath<->Above & Below) : Subsystem
  Inside Enivornment Temperature : Subsystem
      settings: PortSchema="{\"entries\":[{\"content\":{\"sides\":[{\"content\":{\"connectorIds\":[\"LConn1\"]},\"type\":\"ConnectorPlacement.EquallySpacedRectSide\",\"uuid\":\"d7207a88-d4d1-4eb1-8525-bfbf38cfed80\"},{\"content\":{\"connectorIds\":[\"In1\"],\"side\":\"RIGHT\"},\"type\":\"ConnectorPlacement.EquallySpacedRectSide\",\"uuid\":\"a5beddf3-616c-4e89-970e-855bf6dc3854\"},{\"content\":{\"side\":\"TOP\"},\"type\":\"ConnectorPlacement.EquallySpacedRectSide\",\"uuid\":\"3f9b2b25-be8a-4286-a049-e39ed58f5b46\"}]},\"type\":\"ConnectorPlacement.EquallySpacedConnector\",\"uuid\":\"525311df-b3f4-411a-b576-8112a1b0b63b\"}],\"packageUris\":[\"http://schema.mathworks.com/mf0/Connector/R2020b\"],\"version\":\"1.0\"}"
  Outside Temperature : Subsystem
      settings: PortSchema="{\"entries\":[{\"content\":{\"sides\":[{\"content\":{\"connectorIds\":[\"LConn1\"]},\"type\":\"ConnectorPlacement.EquallySpacedRectSide\",\"uuid\":\"d7207a88-d4d1-4eb1-8525-bfbf38cfed80\"},{\"content\":{\"connectorIds\":[\"In1\"],\"side\":\"RIGHT\"},\"type\":\"ConnectorPlacement.EquallySpacedRectSide\",\"uuid\":\"a5beddf3-616c-4e89-970e-855bf6dc3854\"},{\"content\":{\"side\":\"TOP\"},\"type\":\"ConnectorPlacement.EquallySpacedRectSide\",\"uuid\":\"3f9b2b25-be8a-4286-a049-e39ed58f5b46\"}]},\"type\":\"ConnectorPlacement.EquallySpacedConnector\",\"uuid\":\"525311df-b3f4-411a-b576-8112a1b0b63b\"}],\"packageUris\":[\"http://schema.mathworks.com/mf0/Connector/R2020b\"],\"version\":\"1.0\"}"
  SOLAR__WALL : Subsystem
  SOLAR__WINDOW : Subsystem
  TEMP_01 : Subsystem
  Thermal Mass of inside air : fl_lib/Thermal/Thermal Elements/Thermal Mass  mass_type=foundation.enum.constant_variable.constant  mass=P_M_AIR_BATH kg  sp_heat=P_CP_AIR J/(K*kg)  mass_min=1e-6 kg  num_ports=foundation.enum.numPorts2.one  m_specify=off  m_priority=High  m=1 kg  m_nominal_specify=off  m_nominal_unit=kg  m_nominal_value=1  T_specify=on  T_priority=High  T=T_INIT_BDR degC  T_nominal_specify=off  T_nominal_unit=K  T_nominal_value=1  Q_specify=off  Q_priority=None  Q=0 W  Q_nominal_specify=off  Q_nominal_unit=W  Q_nominal_value=1
  Wall (Bath<->Outside) : Subsystem
  Window (Bath<->Outside) : Subsystem
  Conn1 : PMIOPort  Side=Left
  T_BATH : Outport
  wires:
  TEMP_01/1(Sim) -> T_BATH/1
  [T_OUT] -> Outside Temperature/1(T_OUT)
  [T_ENV] -> Inside Enivornment Temperature/1(T_ENV)
  connections:
  Window (Bath<->Outside)/RConn1 -- Outside Temperature/LConn1 -- Wall (Bath<->Outside)/RConn2
  TEMP_01/LConn1 -- Conn1/RConn1 -- Wall (Bath<->Outside)/LConn1 -- Thermal Mass of inside air/LConn1 -- Window (Bath<->Outside)/LConn1 -- Ceiling & Floor (Bath<->Above & Below)/RConn1
  Inside Enivornment Temperature/LConn1 -- Ceiling & Floor (Bath<->Above & Below)/LConn1
  SOLAR__WALL/LConn1 -- Wall (Bath<->Outside)/RConn1
  SOLAR__WINDOW/LConn1 -- Window (Bath<->Outside)/RConn2

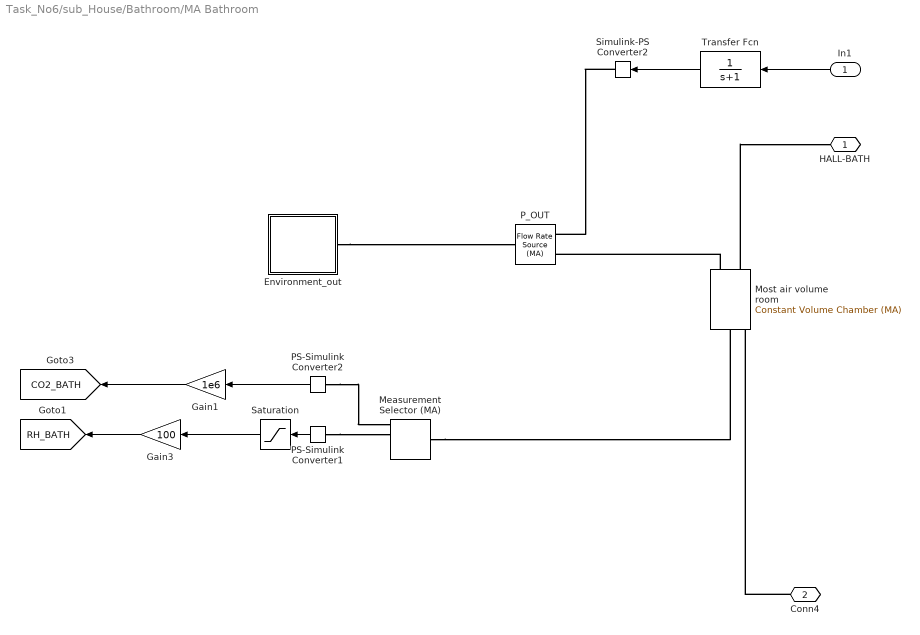
== system Task_No6/sub_House/Bathroom/MA Bathroom ==
  In1 : Inport
  Environment_out : Subsystem
  Gain1 : Gain  Gain=1e6
  Gain3 : Gain  Gain=100
  Measurement Selector (MA) : fl_lib/Moist Air/Sensors/Measurement Selector (MA)  moisture_spec=foundation.enum.moisture_spec.relative_humidity  trace_gas_spec=foundation.enum.trace_gas_spec.mass_fraction
  Most air volume room : fl_lib/Moist Air/Elements/Constant Volume Chamber (MA)  volume=P_M_AIR_BATH/P_DENSITY_AIR m^3  num_ports=foundation.enum.num_ports.two  area_A=P_AREA_DUCT m^2  area_B=P_AREA_SING_DOOR m^2  area_C=0.01 m^2  area_D=0.01 m^2  RH_ws=1  time_constant=1 s  moisture_trace_gas_source=foundation.enum.moisture_trace_gas_source.none  moisture_source_spec=foundation.enum.moisture_source_spec.vapor  moisture_mass_flow=0 kg/s  moisture_temperature_spec=foundation.enum.temperature_spec.atmospheric  moisture_temperature=293.15 K  trace_gas_mass_flow=0 kg/s  trace_gas_temperature_spec=foundation.enum.temperature_spec.atmospheric  trace_gas_temperature=293.15 K  p_I_specify=on  p_I_priority=High  p_I=0.101325 MPa  p_I_nominal_specify=off  p_I_nominal_unit=MPa  p_I_nominal_value=1  T_I_specify=on  T_I_priority=High  T_I=T_INIT_BDR degC  T_I_nominal_specify=off  T_I_nominal_unit=K  T_I_nominal_value=1  RH_I_specify=on  RH_I_priority=High  RH_I=RH_INIT_BDR/100  RH_I_nominal_specify=off  RH_I_nominal_unit=1  RH_I_nominal_value=1  x_w_I_specify=off  x_w_I_priority=None  x_w_I=0  x_w_I_nominal_specify=off  x_w_I_nominal_unit=1  x_w_I_nominal_value=1  y_w_I_specify=off  y_w_I_priority=None  y_w_I=0  y_w_I_nominal_specify=off  y_w_I_nominal_unit=1  y_w_I_nominal_value=1  HR_I_specify=off  HR_I_priority=None  HR_I=0  HR_I_nominal_specify=off  HR_I_nominal_unit=1  HR_I_nominal_value=1  x_g_I_specify=on  x_g_I_priority=High  x_g_I=P_INIT_CO2/1e6  x_g_I_nominal_specify=off  x_g_I_nominal_unit=1  x_g_I_nominal_value=1  y_g_I_specify=off  y_g_I_priority=None  y_g_I=0  y_g_I_nominal_specify=off  y_g_I_nominal_unit=1  y_g_I_nominal_value=1
      settings: InternalSimscapePortConfiguration="{\"Bottom\":[],\"Left\":[{\"id\":\"A\",\"label\":\"A\",\"type\":\"foundation.moist_air.moist_air\"},{\"id\":\"B\",\"label\":\"B\",\"type\":\"foundation.moist_air.moist_air\"}],\"Right\":[{\"id\":\"W\",\"label\":\"W\",\"type\":\"output\"},{\"id\":\"F\",\"label\":\"F\",\"type\":\"output\"},{\"id\":\"H\",\"label\":\"H\",\"type\":\"foundation.thermal.thermal\"}],\"Top\":[]}"
  PS-Simulink Converter1 : nesl_utility/PS-Simulink Converter  PhysicalDomain=network_engine_domain  SubClassName=ps_output  LeftPortType=input  RightPortType=output  PseudoPeriodic=off  Frequencies=[]  VectorFormat=inherit  Unit=inherit  AffineConversion=off
  PS-Simulink Converter2 : nesl_utility/PS-Simulink Converter  PhysicalDomain=network_engine_domain  SubClassName=ps_output  LeftPortType=input  RightPortType=output  PseudoPeriodic=off  Frequencies=[]  VectorFormat=inherit  Unit=inherit  AffineConversion=off
  P_OUT : fl_lib/Moist Air/Sources/Flow Rate Source (MA)  source_type=foundation.enum.constant_controlled.controlled  flow_type=foundation.enum.mass_volumetric_flow.mass  mass_flow=0 kg/s  volumetric_flow=0 m^3/s  volumetric_flow_conditions=foundation.enum.volumetric_flow_conditions.actual  p_std=0.101325 MPa  T_std=20 degC  RH_std=0.65  power_spec=foundation.enum.power_spec.isentropic  area_A=P_AREA_DUCT m^2  area_B=P_AREA_DUCT m^2
      settings: InternalSimscapePortConfiguration="{\"Bottom\":[],\"Left\":[{\"id\":\"A\",\"label\":\"A\",\"type\":\"foundation.moist_air.moist_air\"},{\"id\":\"M\",\"label\":\"M\",\"type\":\"input\"}],\"Right\":[{\"id\":\"B\",\"label\":\"B\",\"type\":\"foundation.moist_air.moist_air\"}],\"Top\":[]}"
  Saturation : Saturate  UpperLimit=1  LowerLimit=0
  Simulink-PS Converter2 : nesl_utility/Simulink-PS Converter  PhysicalDomain=network_engine_domain  SubClassName=ps_input  LeftPortType=input  RightPortType=output  PseudoPeriodic=off  Frequencies=[]  NoiseDistribution=none  NoiseParameters=[]  Unit=1  AffineConversion=off  FilteringAndDerivatives=provide  SimscapeFilterOrder=1  InputFilterTimeConstant=0.001  UdotUserProvided=0
  Transfer Fcn : TransferFcn  Denominator=[1 1]
  HALL-BATH : PMIOPort  Side=Left
  Conn4 : PMIOPort  Port=2  Side=Right
  tag scope: CO2_BATH=global, RH_BATH=global
  wires:
  PS-Simulink Converter1/1 -> Saturation/1
  PS-Simulink Converter2/1 -> Gain1/1
  Saturation/1 -> Gain3/1
  Gain3/1 -> [RH_BATH]
  Gain1/1 -> [CO2_BATH]
  In1/1 -> Transfer Fcn/1
  Transfer Fcn/1 -> Simulink-PS Converter2/1
  connections:
  PS-Simulink Converter1/LConn1 -- Measurement Selector (MA)/RConn3
  PS-Simulink Converter2/LConn1 -- Measurement Selector (MA)/RConn4
  Conn4/RConn1 -- Most air volume room/RConn3
  Measurement Selector (MA)/LConn1 -- Most air volume room/RConn2
  Most air volume room/LConn2 -- HALL-BATH/RConn1
  Most air volume room/LConn1 -- P_OUT/LConn1
  Simulink-PS Converter2/RConn1 -- P_OUT/LConn2
  Environment_out/LConn1 -- P_OUT/RConn1

== system Task_No6/sub_House/Bedroom 1/Bedroom 1 ==
  AirConditioning : Subsystem
  Ceiling & Floor (BDR1<->Above & Below) : Subsystem
  Heat source human : Subsystem
  Inside Enivornment Temperature : Subsystem
      settings: PortSchema="{\"entries\":[{\"content\":{\"sides\":[{\"content\":{\"connectorIds\":[\"LConn1\"]},\"type\":\"ConnectorPlacement.EquallySpacedRectSide\",\"uuid\":\"d7207a88-d4d1-4eb1-8525-bfbf38cfed80\"},{\"content\":{\"connectorIds\":[\"In1\"],\"side\":\"RIGHT\"},\"type\":\"ConnectorPlacement.EquallySpacedRectSide\",\"uuid\":\"a5beddf3-616c-4e89-970e-855bf6dc3854\"},{\"content\":{\"side\":\"TOP\"},\"type\":\"ConnectorPlacement.EquallySpacedRectSide\",\"uuid\":\"3f9b2b25-be8a-4286-a049-e39ed58f5b46\"}]},\"type\":\"ConnectorPlacement.EquallySpacedConnector\",\"uuid\":\"525311df-b3f4-411a-b576-8112a1b0b63b\"}],\"packageUris\":[\"http://schema.mathworks.com/mf0/Connector/R2020b\"],\"version\":\"1.0\"}"
  Outside Temperature : Subsystem
      settings: PortSchema="{\"entries\":[{\"content\":{\"sides\":[{\"content\":{\"connectorIds\":[\"LConn1\"]},\"type\":\"ConnectorPlacement.EquallySpacedRectSide\",\"uuid\":\"d7207a88-d4d1-4eb1-8525-bfbf38cfed80\"},{\"content\":{\"connectorIds\":[\"In1\"],\"side\":\"RIGHT\"},\"type\":\"ConnectorPlacement.EquallySpacedRectSide\",\"uuid\":\"a5beddf3-616c-4e89-970e-855bf6dc3854\"},{\"content\":{\"side\":\"TOP\"},\"type\":\"ConnectorPlacement.EquallySpacedRectSide\",\"uuid\":\"3f9b2b25-be8a-4286-a049-e39ed58f5b46\"}]},\"type\":\"ConnectorPlacement.EquallySpacedConnector\",\"uuid\":\"525311df-b3f4-411a-b576-8112a1b0b63b\"}],\"packageUris\":[\"http://schema.mathworks.com/mf0/Connector/R2020b\"],\"version\":\"1.0\"}"
  SOLAR__WALL : Subsystem
  SOLAR__WINDOW : Subsystem
  TEMP_01 : Subsystem
  Thermal Mass of inside air : fl_lib/Thermal/Thermal Elements/Thermal Mass  mass_type=foundation.enum.constant_variable.constant  mass=P_M_AIR_BDR1 kg  sp_heat=P_CP_AIR J/(K*kg)  mass_min=1e-6 kg  num_ports=foundation.enum.numPorts2.one  m_specify=off  m_priority=High  m=1 kg  m_nominal_specify=off  m_nominal_unit=kg  m_nominal_value=1  T_specify=on  T_priority=High  T=T_INIT_BDR degC  T_nominal_specify=off  T_nominal_unit=K  T_nominal_value=1  Q_specify=off  Q_priority=None  Q=0 W  Q_nominal_specify=off  Q_nominal_unit=W  Q_nominal_value=1
  Wall (BDR1<->Outside) : Subsystem
  Window (BDR1<->Outside) : Subsystem
  Conn1 : PMIOPort  Side=Left
  T_BDR1 : Outport
  wires:
  TEMP_01/1(Sim) -> T_BDR1/1
  [T_OUT] -> Outside Temperature/1(T_OUT)
  [T_ENV] -> Inside Enivornment Temperature/1(T_ENV)
  connections:
  Wall (BDR1<->Outside)/RConn2 -- Outside Temperature/LConn1 -- Window (BDR1<->Outside)/RConn1
  Window (BDR1<->Outside)/LConn1 -- TEMP_01/LConn1 -- AirConditioning/RConn2 -- AirConditioning/RConn1 -- Heat source human/LConn1 -- Conn1/RConn1 -- Wall (BDR1<->Outside)/LConn1 -- Thermal Mass of inside air/LConn1 -- Ceiling & Floor (BDR1<->Above & Below)/RConn1
  Inside Enivornment Temperature/LConn1 -- Ceiling & Floor (BDR1<->Above & Below)/LConn1
  SOLAR__WALL/LConn1 -- Wall (BDR1<->Outside)/RConn1
  SOLAR__WINDOW/LConn1 -- Window (BDR1<->Outside)/RConn2
